simulink model "LabDcMotorDifferentLoad"  (R2020a)
settings: Solver=VariableStepAuto  StartTime=0.0  StopTime=12.0  RelTol=1e-3
libraries: powerlib x4
settings Model: Creator=Samsuzzaman  LastModifiedBy=Samsuzzaman

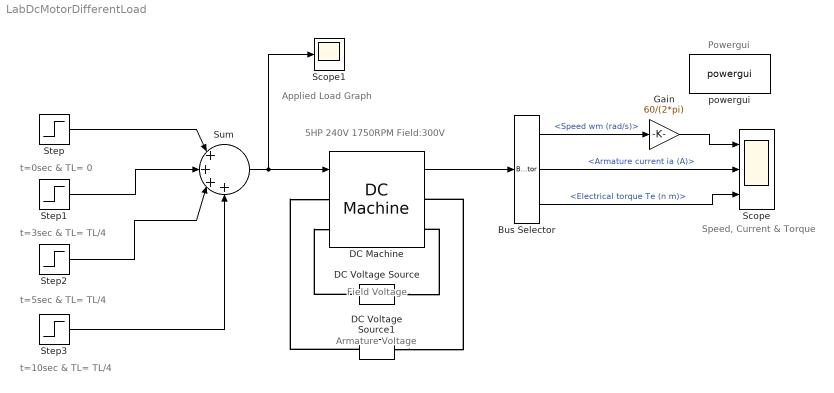
== system LabDcMotorDifferentLoad ==
  note: Speed, Current & Torque
  note: Powergui
  note: Applied Load Graph
  note: Armature Voltage
  note: Field Voltage
  note: t=0sec & TL= 0
  note: 5HP 240V 1750RPM Field:300V
  note: t=3sec & TL= TL/4
  note: t=5sec & TL= TL/4
  note: t=10sec & TL= TL/4
  Bus Selector : BusSelector  OutputSignals=Speed wm (rad/s),Armature current ia (A),Electrical torque Te (n m)
  DC Machine : powerlib/Machines/DC Machine  PresetModel=01: 5HP 240V 1750RPM Field:300V  MechanicalLoad=Torque TL  FieldType=Wound  ShowDetailedParameters=on  MeasurementBus=off  RLa=[2.581 0.028]  RLf=[281.3 156]  Laf=0.9483  MachineConstant=Torque constant (N.m/A)  Ke=1.8  Kt=1.8  J=0.02215  Bm=0.002953  Tf=0.5161  w0=1  Ifinit=1.06647707074298  TsPowergui=0  TsBlock=-1
  DC Voltage Source : powerlib/Electrical Sources/DC Voltage Source  Amplitude=300  Measurements=Voltage
  DC Voltage Source1 : powerlib/Electrical Sources/DC Voltage Source  Amplitude=240  Measurements=Voltage
  Gain : Gain  Gain=60/(2*pi)
  Scope : Scope  NumInputPorts=3
  Scope1 : Scope
  Step : Step  Time=0  After=0  SampleTime=0
  Step1 : Step  Time=3  After=5.09  SampleTime=0
  Step2 : Step  Time=5  After=5.09  SampleTime=0
  Step3 : Step  Time=10  After=5.09  SampleTime=0
  Sum : Sum  Inputs=|++++
  powergui : powerlib/powergui  Priority=1  SimulationMode=Continuous  SampleTime=50e-6  frequency=60  Iterations=50  frequencyindice=0  Pbase=100e6  ErrMax=1e-4  UnitsV=kV  UnitsW=MW  buscounter=0  FunctionMessages=off  echomessages=off  EnableUseOfTLC=off  CurrentSourceSwitches=off  DisableSnubberDevices=off  DisableRonSwitches=off  DisableVfSwitches=off  DisplayEquations=off  AutomaticDiscreteSolvers=off  SolverType=Tustin/Backward Euler (TBE)  Interpol=off  ExternalGateDelay=off  methode=off  Ts=100  x0status=blocks  SPID=on  SwTol=0  HookPort=off  NonlinearTolerance=1e-4  nMaxIteration=100  ContinueOnMaxIteration=off  RestoreLinks=warning  ResistiveCurrentMeasurement=off  Frange=[0:2:500]  Ylog=off  Xlog=on  ShowGrid=off  save=off  variable=ZData  structure=0  ZoomFFT=off  StartTime=0.0  cycles=1  DisplayStyle=1  fundamental=60  FreqAxis=off  MaxFrequency=1000  frequencyindicesteady=1  RmsSteady=1  display=off
  wires:
  Sum/1 -> Scope1/1, DC Machine/1
  Step/1 -> Sum/1
  Step1/1 -> Sum/2
  Step2/1 -> Sum/3
  Step3/1 -> Sum/4
  DC Machine/1 -> Bus Selector/1
  Bus Selector/1 -> Gain/1  "<Speed wm (rad/s)>"
  Bus Selector/2 -> Scope/2  "<Armature current ia (A)>"
  Gain/1 -> Scope/1
  Bus Selector/3 -> Scope/3  "<Electrical torque Te (n m)>"
  connections:
  DC Voltage Source/LConn1 -- DC Machine/RConn2
  DC Voltage Source/RConn1 -- DC Machine/LConn2
  DC Voltage Source1/LConn1 -- DC Machine/RConn1
  DC Voltage Source1/RConn1 -- DC Machine/LConn1
